simulink model "example_of_enable_subsystem"  (R2021a)
settings: Solver=FixedStepAuto  StartTime=0.0  StopTime=10.0  RelTol=1e-3
settings Model: Creator=YasserNet  LastModifiedBy=YasserNet

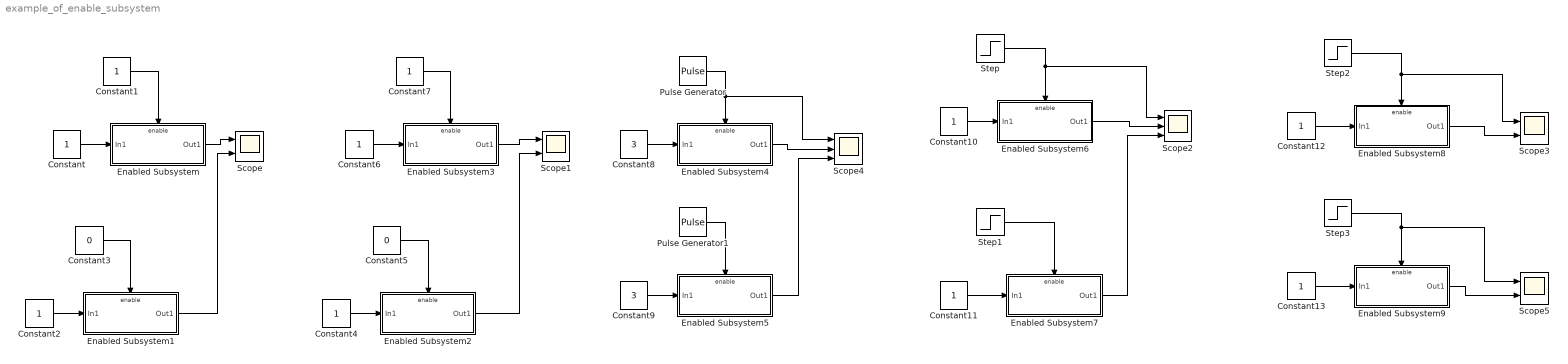
== system example_of_enable_subsystem ==
  Constant{,1..2,4,6..7,10..13} (10 alike) : Constant
  Constant3 : Constant  Value=0
  Constant5 : Constant  Value=0
  Constant8 : Constant  Value=3
  Constant9 : Constant  Value=3
  Enabled Subsystem : Subsystem  TreatAsAtomicUnit=on
  Enabled Subsystem1 : Subsystem  TreatAsAtomicUnit=on
  Enabled Subsystem2 : Subsystem  TreatAsAtomicUnit=on
  Enabled Subsystem3 : Subsystem  TreatAsAtomicUnit=on
  Enabled Subsystem4 : Subsystem  TreatAsAtomicUnit=on
  Enabled Subsystem5 : Subsystem  TreatAsAtomicUnit=on
  Enabled Subsystem6 : Subsystem  TreatAsAtomicUnit=on
  Enabled Subsystem7 : Subsystem  TreatAsAtomicUnit=on
  Enabled Subsystem8 : Subsystem  TreatAsAtomicUnit=on
  Enabled Subsystem9 : Subsystem  TreatAsAtomicUnit=on
  Pulse Generator : DiscretePulseGenerator  PulseType=Time based  PulseWidth=50
  Pulse Generator1 : DiscretePulseGenerator  PulseType=Time based  PulseWidth=50
  Scope{,1,3,5} (4 alike) : Scope  NumInputPorts=2
  Scope2 : Scope  NumInputPorts=3
  Scope4 : Scope  NumInputPorts=3
  Step : Step  SampleTime=0
  Step1 : Step  SampleTime=0
  Step2 : Step  Time=0  Before=-1  After=0  SampleTime=0
  Step3 : Step  Time=0  Before=1  After=2  SampleTime=0
  wires:
  Constant/1 -> Enabled Subsystem/1(In1)
  Constant1/1 -> Enabled Subsystem/Enable
  Enabled Subsystem/1(Out1) -> Scope/1
  Enabled Subsystem1/1(Out1) -> Scope/2
  Constant3/1 -> Enabled Subsystem1/Enable
  Constant2/1 -> Enabled Subsystem1/1(In1)
  Constant4/1 -> Enabled Subsystem2/1(In1)
  Constant5/1 -> Enabled Subsystem2/Enable
  Enabled Subsystem3/1(Out1) -> Scope1/1
  Constant7/1 -> Enabled Subsystem3/Enable
  Constant6/1 -> Enabled Subsystem3/1(In1)
  Constant8/1 -> Enabled Subsystem4/1(In1)
  Pulse Generator/1 -> Scope4/1, Enabled Subsystem4/Enable
  Enabled Subsystem4/1(Out1) -> Scope4/2
  Enabled Subsystem2/1(Out1) -> Scope1/2
  Enabled Subsystem5/1(Out1) -> Scope4/3
  Pulse Generator1/1 -> Enabled Subsystem5/Enable
  Constant9/1 -> Enabled Subsystem5/1(In1)
  Enabled Subsystem6/1(Out1) -> Scope2/2
  Step/1 -> Scope2/1, Enabled Subsystem6/Enable
  Constant10/1 -> Enabled Subsystem6/1(In1)
  Constant11/1 -> Enabled Subsystem7/1(In1)
  Step1/1 -> Enabled Subsystem7/Enable
  Enabled Subsystem7/1(Out1) -> Scope2/3
  Enabled Subsystem8/1(Out1) -> Scope3/2
  Step2/1 -> Scope3/1, Enabled Subsystem8/Enable
  Constant12/1 -> Enabled Subsystem8/1(In1)
  Constant13/1 -> Enabled Subsystem9/1(In1)
  Step3/1 -> Scope5/1, Enabled Subsystem9/Enable
  Enabled Subsystem9/1(Out1) -> Scope5/2

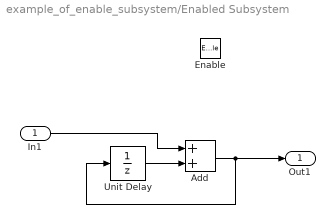
== system example_of_enable_subsystem/Enabled Subsystem ==
  In1 : Inport
  Enable : EnablePort
  Add : Sum
  Unit Delay : UnitDelay  HasFrameUpgradeWarning=on
  Out1 : Outport
  wires:
  In1/1 -> Add/1
  Add/1 -> Out1/1, Unit Delay/1
  Unit Delay/1 -> Add/2

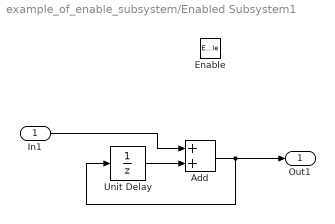
== system example_of_enable_subsystem/Enabled Subsystem1 ==
  In1 : Inport
  Enable : EnablePort
  Add : Sum
  Unit Delay : UnitDelay  HasFrameUpgradeWarning=on
  Out1 : Outport
  wires:
  Unit Delay/1 -> Add/2
  Add/1 -> Unit Delay/1, Out1/1
  In1/1 -> Add/1

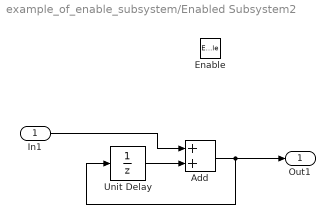
== system example_of_enable_subsystem/Enabled Subsystem2 ==
  In1 : Inport
  Enable : EnablePort  StatesWhenEnabling=reset
  Add : Sum
  Unit Delay : UnitDelay  HasFrameUpgradeWarning=on
  Out1 : Outport
  wires:
  In1/1 -> Add/1
  Add/1 -> Out1/1, Unit Delay/1
  Unit Delay/1 -> Add/2

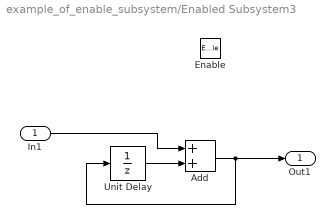
== system example_of_enable_subsystem/Enabled Subsystem3 ==
  In1 : Inport
  Enable : EnablePort  StatesWhenEnabling=reset
  Add : Sum
  Unit Delay : UnitDelay  HasFrameUpgradeWarning=on
  Out1 : Outport
  wires:
  Unit Delay/1 -> Add/2
  Add/1 -> Unit Delay/1, Out1/1
  In1/1 -> Add/1

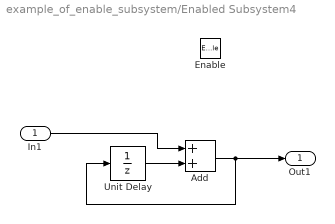
== system example_of_enable_subsystem/Enabled Subsystem4 ==
  In1 : Inport
  Enable : EnablePort  StatesWhenEnabling=reset
  Add : Sum
  Unit Delay : UnitDelay  SampleTime=-1  HasFrameUpgradeWarning=on
  Out1 : Outport
  wires:
  In1/1 -> Add/1
  Add/1 -> Out1/1, Unit Delay/1
  Unit Delay/1 -> Add/2

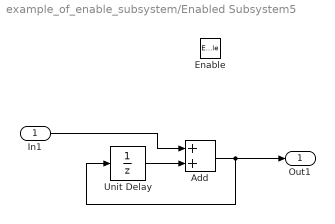
== system example_of_enable_subsystem/Enabled Subsystem5 ==
  In1 : Inport
  Enable : EnablePort
  Add : Sum
  Unit Delay : UnitDelay  SampleTime=-1  HasFrameUpgradeWarning=on
  Out1 : Outport
  wires:
  Unit Delay/1 -> Add/2
  Add/1 -> Unit Delay/1, Out1/1
  In1/1 -> Add/1

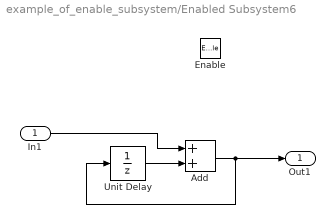
== system example_of_enable_subsystem/Enabled Subsystem6 ==
  In1 : Inport
  Enable : EnablePort  StatesWhenEnabling=reset
  Add : Sum
  Unit Delay : UnitDelay  SampleTime=-1  HasFrameUpgradeWarning=on
  Out1 : Outport
  wires:
  Unit Delay/1 -> Add/2
  Add/1 -> Unit Delay/1, Out1/1
  In1/1 -> Add/1

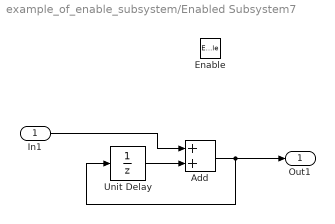
== system example_of_enable_subsystem/Enabled Subsystem7 ==
  In1 : Inport
  Enable : EnablePort
  Add : Sum
  Unit Delay : UnitDelay  SampleTime=-1  HasFrameUpgradeWarning=on
  Out1 : Outport
  wires:
  In1/1 -> Add/1
  Add/1 -> Out1/1, Unit Delay/1
  Unit Delay/1 -> Add/2

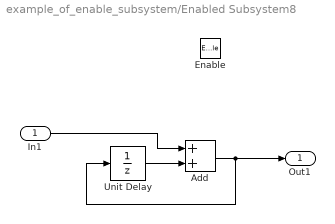
== system example_of_enable_subsystem/Enabled Subsystem8 ==
  In1 : Inport
  Enable : EnablePort
  Add : Sum
  Unit Delay : UnitDelay  HasFrameUpgradeWarning=on
  Out1 : Outport
  wires:
  Unit Delay/1 -> Add/2
  Add/1 -> Unit Delay/1, Out1/1
  In1/1 -> Add/1

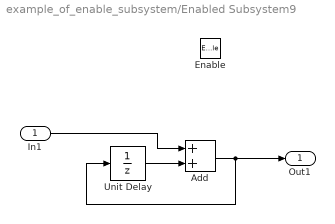
== system example_of_enable_subsystem/Enabled Subsystem9 ==
  In1 : Inport
  Enable : EnablePort
  Add : Sum
  Unit Delay : UnitDelay  HasFrameUpgradeWarning=on
  Out1 : Outport
  wires:
  In1/1 -> Add/1
  Add/1 -> Out1/1, Unit Delay/1
  Unit Delay/1 -> Add/2
